simulink model "tqdtqr_rebuild_V3"  (R2021b)
settings: Solver=VariableStepAuto  StartTime=0.0  StopTime=10.0  RelTol=1e-3
undefined symbols (not defined in the file): ATQD_AfterTqMinGain_X_Deg, ATQD_APSCreepBaseTqD_X_kph, ATQD_APSCreepBaseTqD_Y_Deg, ATQD_APSCreepBaseTqR_X_kph, ATQD_APSCreepBaseTqR_Y_Deg, ATQD_APSCreepIterm_X_kph, ATQD_APSCreepIterm_Y_kph, ATQD_APSCreepPterm_X_kph, ATQD_APSCreepPterm_Y_kph, ATQD_APSDecReq_X_kph, ATQD_APSDecReq_Y_mps2, ATQD_APSDecReqCMD_X_kph, ATQD_APSDecReqTs_X_pct, ATQD_APSDecTimeGain_X_Deg, ATQD_APSDecTimeGain_Y_s, ATQD_APSReqLowSpd_X_Deg, ATQD_AutoHoldReleaseBPS_X_Deg, ATQD_AWDLoadTrqnsGain_X_kg, ATQD_AWDLoadTrqnsGain_Y_pct, ATQD_BOSEnBPSPosn_X_kph, ATQD_BOSMap_X_rpm, ATQD_BOSMap_Y_pct, ATQD_CreepBaseTqD_X_kph, ATQD_CreepBaseTqD_Y_Deg, ATQD_CreepBaseTqR_X_kph, ATQD_CreepBaseTqR_Y_Deg, ATQD_CreepBPSDisPosn_X_Deg, ATQD_CreepBPSDisPosnR_X_Deg, ATQD_CreepBPSEnPosn_X_Deg, ATQD_CreepBPSEnPosnR_X_Deg, ATQD_CreepDeltaTq_X_kph, ATQD_CreepIterm_X_kph, ATQD_CreepIterm_Y_kph, ATQD_CreepItermMaxLimit_X_pct, ATQD_CreepPreloadTime_X_kph, ATQD_CreepPreloadTq_X_kph, ATQD_CreepPreloadTq_Y_s, ATQD_CreepProtTq_X_Deg, ATQD_CreepPterm_X_kph, ATQD_CreepPterm_Y_kph, ATQD_CreepRrTqSpRat_X_rpm, ATQD_CreepRrTqSpRat_Y_Nm, ATQD_CreepTargetSpdD_X_pct, ATQD_CreepTargetSpdR_X_pct, ATQD_CreepUpLimitTq_X_rpm, ATQD_DecIneOPDHoldEnDelay_X_Deg, ATQD_DecIneOPDHoldEnDelay_Y_bar, ATQD_ECOTqMapD_X_rpm, ATQD_ECOTqMapD_Y_pct, ATQD_EMTqMapD_X_rpm, ATQD_EMTqMapD_Y_pct, ATQD_EOPDTqMapDCon_X_rpm, ATQD_EOPDTqMapDCon_Y_Deg, ATQD_EstInitVehWeight_X_c, ATQD_FAfterTqCMDGain_X_rpm, ATQD_FAfterTqCMDGain_Y_pct, ATQD_ForceLowSpd_X_Deg, ATQD_ForcePLimitSpd_X_Deg, ATQD_FrLossMAPLowV_X_rpm, ATQD_FrLossMAPLowV_Y_Nm ... (+949)
libraries: simulink x235, hcu_lib x208, tqr x63, tqd x6
(part 24 of 37)

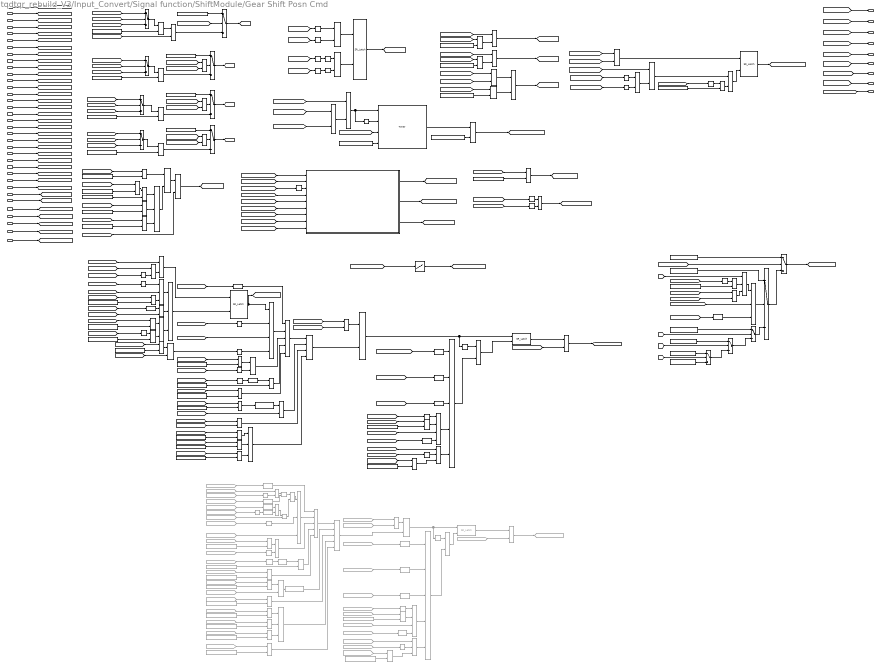
== system tqdtqr_rebuild_V3/Input_Convert/Signal function/ShiftModule/Gear Shift Posn Cmd ==
  note: Get max wheel rpm
  note: Allow D R conditions
  note: Prevent user accidental touch D to N
  note: Force P conditions
  note: Allow P N conditions
  note: Decide final gear shifter CMD
  note: Shifter value determine with DDM detection
  note: Failsafe for Shifter PButton fail
  VTQD_ShifterHandleCmd_enum : Inport
  VPMM_PowerSta_enum : Inport  Port=2
  VINP_DrDoorSW_flg : Inport  Port=3
  VVMC_APSShiftPosnReq_enum : Inport  Port=4
  VVMC_APSActive_flg : Inport  Port=5
  VINP_DriverSeatBeltCmd_flg : Inport  Port=6
  VTQD_EPBCarWashMode_flg : Inport  Port=7
  VTQD_VehActSpd_kph : Inport  Port=8
  VINP_ChrgPlugSta_enum : Inport  Port=9
  VTQD_GearActualPosn_enum : Inport  Port=10
  VTQD_AfterAvailableTqDemFr_Nm : Inport  Port=11
  VTQD_AfterAvailableTqDemRr_Nm : Inport  Port=12
  VTQR_NoABSFEDUWhlTqReq_Nm : Inport  Port=13
  VTQR_NoABSREDUWhlTqReq_Nm : Inport  Port=14
  task_time_s : Inport  Port=15
  VINP_DOASta_flg : Inport  Port=16
  VTQD_IVIPwrLock_flg : Inport  Port=17
  VTQD_BrkSwSta_flg : Inport  Port=18
  VTQD_OPDHoldAllowPark_flg : Inport  Port=19
  VINP_CAASSta_enum : Inport  Port=20
  VDDM_VCURAPSErrLv2_flg : Inport  Port=21
  VDDM_VCURAPSErrLv3_flg : Inport  Port=22
  VINP_APSStaSystem_enum : Inport  Port=23
  VDDM_Shifter1Err_flg : Inport  Port=24
  SWC_RegenUp : Inport  Port=25
  SWC_RegenDown : Inport  Port=26
  VDDM_ShifterSigErrCFS_flg : Inport  Port=27
  VTQD_ShifterFailsta_enum : Inport  Port=28
  VTQD_FrShaftSpd_rpm : Inport  Port=29
  VTQD_RrShaftSpd_rpm : Inport  Port=30
  VINP_EPBSta_enum : Inport  Port=31
  VINP_VehSpeed_kph : Inport  Port=32
  VVMC_EstSlope_Deg : Inport  Port=33
  VPMM_DrSeatSta_enum : Inport  Port=34
  VINP_ShifterHandleCmd_enum : Inport  Port=35
  AND : Logic  Commented=on  AllPortsSameDT=off  OutDataTypeStr=boolean
  AND1 : Logic  Commented=on  AllPortsSameDT=off  OutDataTypeStr=boolean
  AND{6,8..12,14..15,21..22} (10 alike) : Logic  AllPortsSameDT=off  OutDataTypeStr=boolean
  AND13 : Logic  Inputs=3  AllPortsSameDT=off  OutDataTypeStr=boolean
  AND16 : Logic  Inputs=4  AllPortsSameDT=off  OutDataTypeStr=boolean
  AND17 : Logic  Operator=OR  AllPortsSameDT=off  OutDataTypeStr=boolean
  AND18 : Logic  Inputs=4  AllPortsSameDT=off  OutDataTypeStr=boolean
  AND19 : Logic  Inputs=4  AllPortsSameDT=off  OutDataTypeStr=boolean
  AND2 : Logic  Commented=on  Inputs=4  AllPortsSameDT=off  OutDataTypeStr=boolean
  AND20 : Logic  Operator=OR  AllPortsSameDT=off  OutDataTypeStr=boolean
  AND3 : Logic  Commented=on  Operator=OR  AllPortsSameDT=off  OutDataTypeStr=boolean
  AND4 : Logic  Commented=on  Inputs=3  AllPortsSameDT=off  OutDataTypeStr=boolean
  AND5 : Logic  Commented=on  Inputs=5  AllPortsSameDT=off  OutDataTypeStr=boolean
  AND7 : Logic  Commented=on  AllPortsSameDT=off  OutDataTypeStr=boolean
  Constant : Constant  Value=ENUM_GEARSHIFTCMD_R
  Constant1 : Constant  Value=ENUM_POWERSTA_READY
  Constant10 : Constant  Value=KTQD_StandbyAllowPNSW_flg
  Constant11 : Constant  Commented=on  Value=KTQD_OPDHoldAllowGearPSW_flg
  Constant12 : Constant  Value=ENUM_SHIFTCOMMAND_D
  Constant13 : Constant  Value=ENUM_SHIFTCOMMAND_N
  Constant14 : Constant  Commented=on  Value=ENUM_CAASSTA_SHIFTGEARTOP
  Constant15 : Constant  Commented=on  Value=ENUM_PWRSTASW_READY
  Constant16 : Constant  Commented=on  Value=ENUM_SHIFTCOMMAND_P
  Constant17 : Constant  Value=ENUM_POWERSTA_STANDBY
  Constant18 : Constant  Value=ENUM_POWERSTA_ON
  Constant19 : Constant  Value=ENUM_POWERSTA_READY
  Constant2 : Constant  Value=ENUM_GEARSHIFTCMD_N
  Constant20 : Constant  Commented=on  Value=ENUM_CHRGPLUGSTA_NONE
  Constant21 : Constant  Commented=on  Value=ENUM_APSSYSTEMSTA_REMOTEACTIVE
  Constant22 : Constant  Value=ENUM_CHRGPLUGSTA_NONE
  Constant23 : Constant  Commented=on  Value=ENUM_APSSYSTEMSTA_REMOTEACTIVE
  Constant24 : Constant  Commented=on  Value=ENUM_PWRSTASW_STANDBY
  Constant25 : Constant  Commented=on  Value=ENUM_PWRSTASW_ON
  Constant26 : Constant  Commented=on  Value=ENUM_PWRSTASW_READY
  Constant27 : Constant  Value=KTQD_ShifterFail2P_s
  Constant28 : Constant  Value=KTQD_ShifterFail2P_s
  Constant29 : Constant  Value=KTQD_ForcePLimitSpd_kph
  Constant3 : Constant  Value=ENUM_GEARSHIFTCMD_P
  Constant30 : Constant  Value=ENUM_SHIFTERERRSTA_PBUTTONFAILURE
  Constant31 : Constant  Value=ENUM_SHIFTERERRSTA_HALLFAILURE
  Constant{5,32..34} (4 alike) : Constant  Value=FALSE
  Constant35 : Constant  Value=ENUM_SHIFTERERRSTA_SHIFTERFAILURE
  Constant36 : Constant  Value=ENUM_SHIFTCOMMAND_R
  Constant37 : Constant  Commented=on  Value=KTQD_ForcePLimitSpd_kph
  Constant38 : Constant  Value=KTQD_OPDHoldAllowGearPSW_flg
  Constant39 : Constant  Value=ENUM_CAASSTA_SHIFTGEARTOP
  Constant4 : Constant  Value=ENUM_GEARSHIFTCMD_D
  Constant40 : Constant  Value=ENUM_PWRSTASW_READY
  Constant41 : Constant  Value=ENUM_SHIFTCOMMAND_P
  Constant42 : Constant  Value=ENUM_CHRGPLUGSTA_NONE
  Constant43 : Constant  Value=ENUM_APSSYSTEMSTA_REMOTEACTIVE
  Constant44 : Constant  Value=ENUM_APSSYSTEMSTA_REMOTEACTIVE
  Constant45 : Constant  Value=ENUM_PWRSTASW_STANDBY
  Constant46 : Constant  Value=ENUM_PWRSTASW_ON
  Constant47 : Constant  Value=ENUM_PWRSTASW_READY
  Constant48 : Constant  Value=ENUM_EPBSTA_APPLIED
  Constant49 : Constant  Value=KTQD_DoorOpen2GearPRestSpd_kph
  Constant50 : Constant  Value=ENUM_GEARACTUALPOSN_P
  Constant6 : Constant  Value=ENUM_GEARSHIFTCMD_NONE
  Constant7 : Constant  Value=ENUM_GEARSHIFTCMD_P
  Constant8 : Constant  Value=ENUM_SHIFTCOMMAND_P
  Constant9 : Constant  Value=KTQD_DriveProtVehSpdGain_kph
  Delay : Delay  Commented=on  DelayLength=1
  Delay1 : Delay  Commented=on  DelayLength=1
  Delay{4..6,10..11} (5 alike) : Delay  DelayLength=1  InitialCondition=single(0)
      settings: AttributesFormatString=%<InitialCondition>
  Delay{2..3,7..8,12..13} (6 alike) : Delay  DelayLength=1
  Delay9 : Delay  DelayLength=1  InitialCondition=ENUM_GEARACTUALPOSN_P
      settings: AttributesFormatString=%<InitialCondition>
  Detect Change : simulink/Logic and Bit Operations/Detect Change  Commented=on  vinit=uint8(0)  OutDataTypeStr=boolean
  Detect Change1 : simulink/Logic and Bit Operations/Detect Change  Commented=on  vinit=uint8(0)  OutDataTypeStr=boolean
  Detect Change2 : simulink/Logic and Bit Operations/Detect Change  vinit=0  OutDataTypeStr=boolean
  Detect Change3 : simulink/Logic and Bit Operations/Detect Change  vinit=0  OutDataTypeStr=boolean
  Detect Change4 : simulink/Logic and Bit Operations/Detect Change  vinit=boolean(0)  OutDataTypeStr=boolean
  Detect Decrease1 : simulink/Logic and Bit Operations/Detect Decrease  Commented=on  vinit=0.0  OutDataTypeStr=boolean
  Detect Decrease2 : simulink/Logic and Bit Operations/Detect Decrease  vinit=0.0  OutDataTypeStr=boolean
  Detect Increase : simulink/Logic and Bit Operations/Detect Increase  vinit=boolean(0)  OutDataTypeStr=boolean
  Detect Increase{1..5} (5 alike) : simulink/Logic and Bit Operations/Detect Increase  Commented=on  vinit=boolean(0)  OutDataTypeStr=boolean
  Detect Increase6 : simulink/Logic and Bit Operations/Detect Increase  Commented=on  vinit=0.0  OutDataTypeStr=boolean
  Detect Increase7 : simulink/Logic and Bit Operations/Detect Increase  vinit=0.0  OutDataTypeStr=boolean
  Detect Increase8 : simulink/Logic and Bit Operations/Detect Increase  vinit=0.0  OutDataTypeStr=boolean
  Detect Increase9 : simulink/Logic and Bit Operations/Detect Increase  vinit=0.0  OutDataTypeStr=boolean
  Drive Protection : Subsystem
  Equal{,1..2,4..7,9,16..20,22..23,25..26} (17 alike) : RelationalOperator  Operator===  OutDataTypeStr=boolean  RndMeth=Simplest
  Equal{3,10,12..13,15} (5 alike) : RelationalOperator  Commented=on  Operator===  OutDataTypeStr=boolean  RndMeth=Simplest
  Equal11 : RelationalOperator  Commented=on  Operator=~=  OutDataTypeStr=boolean  RndMeth=Simplest
  Equal14 : RelationalOperator  Commented=on  Operator=~=  OutDataTypeStr=boolean  RndMeth=Simplest
  Equal21 : RelationalOperator  Operator=~=  OutDataTypeStr=boolean  RndMeth=Simplest
  Equal24 : RelationalOperator  Operator=~=  OutDataTypeStr=boolean  RndMeth=Simplest
  Equal8 : RelationalOperator  Operator=<=  OutDataTypeStr=boolean  RndMeth=Simplest
  From{27,46,53,108} (4 alike) : From  Commented=on  GotoTag=VTQD_EPBCarWashMode_flg
  From12 : From  Commented=on  GotoTag=VINP_DOASta_flg
  From13 : From  Commented=on  GotoTag=VTQD_ShifterHandleCmd_enum
  From26 : From  Commented=on  GotoTag=VTQD_IVIPwrLock_flg
  From28 : From  Commented=on  GotoTag=VVMC_APSActive_flg
  From32 : From  Commented=on  GotoTag=VTQD_OPDHoldAllowPark_flg
  From42 : From  Commented=on  GotoTag=VINP_CAASSta_enum
  From43 : From  Commented=on  GotoTag=VINP_DrDoorSW_flg
  From44 : From  Commented=on  GotoTag=VINP_SeatSW_flg
  From45 : From  Commented=on  GotoTag=VINP_DriverSeatBeltCmd_flg
  From47 : From  Commented=on  GotoTag=VTQD_VehActSpd_kph
  From48 : From  Commented=on  GotoTag=VINP_ChrgPlugSta_enum
  From{49..52} (4 alike) : From  Commented=on  GotoTag=VPMM_PowerSta_enum
  From54 : From  Commented=on  GotoTag=VINP_DrDoorSW_flg
  From55 : From  Commented=on  GotoTag=VINP_SeatSW_flg
  From56 : From  Commented=on  GotoTag=VINP_DriverSeatBeltCmd_flg
  From57 : From  Commented=on  GotoTag=VTQD_ForceP_flg
  From58 : From  Commented=on  GotoTag=VVMC_APSShiftPosnReq_enum
  From59 : From  Commented=on  GotoTag=VVMC_APSActive_flg
  From60 : From  Commented=on  GotoTag=VVMC_APSShiftPosnReq_enum
  From61 : From  Commented=on  GotoTag=VDDM_VCURAPSErrLv2_flg
  From62 : From  Commented=on  GotoTag=VDDM_VCURAPSErrLv3_flg
  From63 : From  Commented=on  GotoTag=VDDM_VCURAPSErrLv3_flg
  From64 : From  Commented=on  GotoTag=VINP_APSStaSystem_enum
  From65 : From  Commented=on  GotoTag=VINP_DOASta_flg
  From66 : From  Commented=on  GotoTag=VVMC_APSActive_flg
  From69 : From  Commented=on  GotoTag=VINP_APSStaSystem_enum
  Goto22 : Goto  Commented=on  GotoTag=VTQD_ForceP_flg
  Latch : hcu_lib/Basic_Blocks/Latch  Commented=on
  Latch1 : hcu_lib/Basic_Blocks/Latch
  Logical Operator : Logic  Commented=on  AllPortsSameDT=off  OutDataTypeStr=boolean
  Logical Operator1 : Logic  Commented=on  AllPortsSameDT=off  OutDataTypeStr=boolean
  Logical Operator{10..12,14,20,23,25,27} (8 alike) : Logic  AllPortsSameDT=off  OutDataTypeStr=boolean
      Logical Operator20 settings: AttributesFormatString=%<Operator>
  Logical Operator{8..9,13,16..19,24} (8 alike) : Logic  Operator=OR  AllPortsSameDT=off  OutDataTypeStr=boolean
      Logical Operator24 settings: AttributesFormatString=%<Operator>
  Logical Operator{5,15,21..22} (4 alike) : Logic  Operator=NOT  AllPortsSameDT=off  OutDataTypeStr=boolean
  Logical Operator2 : Logic  Inputs=3  AllPortsSameDT=off  OutDataTypeStr=boolean
  Logical Operator26 : Logic  Inputs=3  AllPortsSameDT=off  OutDataTypeStr=boolean
  Logical Operator3 : Logic  Operator=OR  Inputs=3  AllPortsSameDT=off  OutDataTypeStr=boolean
  Logical Operator4 : Logic  Commented=on  Operator=NOT  AllPortsSameDT=off  OutDataTypeStr=boolean
  Logical Operator6 : Logic  Commented=on  Inputs=3  AllPortsSameDT=off  OutDataTypeStr=boolean
  Logical Operator7 : Logic  Commented=on  AllPortsSameDT=off  OutDataTypeStr=boolean
  MTQD_ForcePLimitSpd_Y_kph : Lookup_n-D  NumberOfTableDimensions=1  BreakpointsForDimension1=ATQD_ForcePLimitSpd_X_Deg  Table=MTQD_ForcePLimitSpd_Y_kph  ExtrapMethod=Clip  InternalRulePriority=Speed  RndMeth=Simplest  InputSameDT=on
  Max : MinMax  Function=max  Inputs=2
  NOT{,2..5} (5 alike) : Logic  Commented=on  Operator=NOT  AllPortsSameDT=off  OutDataTypeStr=boolean
  NOT{1,6..12} (8 alike) : Logic  Operator=NOT  AllPortsSameDT=off  OutDataTypeStr=boolean
  OR : Logic  Operator=OR  Inputs=3  AllPortsSameDT=off  OutDataTypeStr=boolean
  OR1 : Logic  Commented=on  Operator=OR  Inputs=5  AllPortsSameDT=off  OutDataTypeStr=boolean
  OR{2,5..6,9..10} (5 alike) : Logic  Commented=on  Operator=OR  AllPortsSameDT=off  OutDataTypeStr=boolean
  OR11 : Logic  Operator=OR  Inputs=5  AllPortsSameDT=off  OutDataTypeStr=boolean
  OR{3..4,12..13} (4 alike) : Logic  Operator=OR  AllPortsSameDT=off  OutDataTypeStr=boolean
  OR14 : Logic  Operator=OR  Inputs=3  AllPortsSameDT=off  OutDataTypeStr=boolean
  OR15 : Logic  Operator=OR  Inputs=5  AllPortsSameDT=off  OutDataTypeStr=boolean
  OR16 : Logic  Operator=OR  Inputs=3  AllPortsSameDT=off  OutDataTypeStr=boolean
  OR7 : Logic  Commented=on  Operator=OR  Inputs=5  AllPortsSameDT=off  OutDataTypeStr=boolean
  OR8 : Logic  Commented=on  Operator=OR  Inputs=3  AllPortsSameDT=off  OutDataTypeStr=boolean
  Relational Operator{,6,8,10} (4 alike) : RelationalOperator  Operator===  OutDataTypeStr=boolean  RndMeth=Simplest
  Relational Operator1 : RelationalOperator  Commented=on  Operator===  OutDataTypeStr=boolean  RndMeth=Simplest
  Relational Operator2 : RelationalOperator  Commented=on  Operator=<=  OutDataTypeStr=boolean  RndMeth=Simplest
  Relational Operator3 : RelationalOperator  OutDataTypeStr=boolean  RndMeth=Simplest
  Relational Operator4 : RelationalOperator  Operator=<=  OutDataTypeStr=boolean  RndMeth=Simplest
  Relational Operator5 : RelationalOperator  Commented=on  Operator=~=  OutDataTypeStr=boolean  RndMeth=Simplest
  Relational Operator7 : RelationalOperator  Operator=<=  OutDataTypeStr=boolean  RndMeth=Simplest
  Relational Operator9 : RelationalOperator  Operator=>  OutDataTypeStr=boolean  RndMeth=Simplest
  SR_Latch{,2..4} (4 alike) : hcu_lib/Basic_Blocks/SR_Latch
  SR_Latch1 : hcu_lib/Basic_Blocks/SR_Latch  Commented=on
  Switch{,1..12} (13 alike) : Switch  Criteria=u2 ~= 0
      settings: AttributesFormatString=%<Criteria>
  Timer : hcu_lib/Basic_Blocks/Timer
  VTQD_GearShiftCMD_enum : Outport
  VTQD_PwrStaAllowPN_flg : Outport  Port=2
  VTQD_PwrStaAllowDR_flg : Outport  Port=3
  VTQD_DriveProtRemove_flg : Outport  Port=4
  VTQD_DriveProtEn_flg : Outport  Port=5
  VTQD_ForceP_flg : Outport  Port=6
  VTQD_MaxShaftSpd_rpm : Outport  Port=7
  VTQD_DOALatchReq_flg : Outport  Port=8
  VTQD_ForcePLimitSpd_kph : Outport  Port=9
  wires:
  Switch2/1 -> Switch4/3
  Constant2/1 -> Switch4/1
  Switch1/1 -> Switch2/3
  [P] -> Switch2/2
  Constant3/1 -> Switch2/1
  Switch3/1 -> Switch1/3
  Constant/1 -> Switch3/1
  Constant4/1 -> Switch1/1
  [R] -> Switch3/2
  [D] -> Switch1/2
  VTQD_ShifterHandleCmd_enum/1 -> [VTQD_ShifterHandleCmd_enum]
  VPMM_PowerSta_enum/1 -> [VPMM_PowerSta_enum]
  [VPMM_PowerSta_enum] -> Equal7/1
  Constant1/1 -> Equal7/2
  Constant6/1 -> Switch3/3
  Switch4/1 -> Switch/3
  VINP_DrDoorSW_flg/1 -> [VINP_DrDoorSW_flg]
  [VTQD_ForceP_flg] -> Switch/2
  Constant7/1 -> Switch/1
  VVMC_APSShiftPosnReq_enum/1 -> [VVMC_APSShiftPosnReq_enum]
  VVMC_APSActive_flg/1 -> [VVMC_APSActive_flg]
  VINP_DriverSeatBeltCmd_flg/1 -> [VINP_DriverSeatBeltCmd_flg]
  VTQD_EPBCarWashMode_flg/1 -> [VTQD_EPBCarWashMode_flg]
  VINP_ChrgPlugSta_enum/1 -> [VINP_ChrgPlugSta_enum]
  VTQR_NoABSREDUWhlTqReq_Nm/1 -> [VTQR_NoABSREDUWhlTqReq_Nm]
  VTQD_AfterAvailableTqDemFr_Nm/1 -> [VTQD_AfterAvailableTqDemFr_Nm]
  VTQD_GearActualPosn_enum/1 -> [VTQD_GearActualPosn_enum]
  VTQR_NoABSFEDUWhlTqReq_Nm/1 -> [VTQR_NoABSFEDUWhlTqReq_Nm]
  VTQD_AfterAvailableTqDemRr_Nm/1 -> [VTQD_AfterAvailableTqDemRr_Nm]
  task_time_s/1 -> [task_time_s]
  VINP_DOASta_flg/1 -> [VINP_DOASta_flg]
  Constant9/1 -> Equal8/2
  [VTQD_VehActSpd_kph] -> Delay11/1
  [VTQD_EPBCarWashMode_flg] -> Detect Increase/1
  Detect Increase/1 -> Logical Operator3/3
  [N] -> Logical Operator2/1
  Logical Operator2/1 -> Logical Operator3/1
  Logical Operator3/1 -> Switch4/2
  [task_time_s] -> Drive Protection/8(task_time_s)  "task_time_s"
  [VTQD_VehActSpd_kph] -> Delay6/1
  [VTQD_AfterAvailableTqDemRr_Nm] -> Drive Protection/7(VTQD_AfterAvailableTqDemRr_Nm)
  [VTQD_AfterAvailableTqDemFr_Nm] -> Drive Protection/4(VTQD_AfterAvailableTqDemFr_Nm)
  [VTQR_NoABSREDUWhlTqReq_Nm] -> Drive Protection/5(VTQR_NoABSREDUWhlTqReq_Nm)
  [VTQR_NoABSFEDUWhlTqReq_Nm] -> Drive Protection/6(VTQR_NoABSFEDUWhlTqReq_Nm)
  [VTQD_ShifterHandleCmd_enum] -> Drive Protection/1(VTQD_ShifterHandleCmd_enum)
  Drive Protection/2(VTQD_DriveProtToPsnN_flg) -> [VTQD_DriveProtToPsnN_flg]
  [VTQD_GearActualPosn_enum] -> Drive Protection/2(VTQD_GearActualPosn_enum)
  VTQD_IVIPwrLock_flg/1 -> [VTQD_IVIPwrLock_flg]
  [VTQD_DriveProtToPsnN_flg] -> Logical Operator3/2
  Equal8/1 -> Logical Operator2/2
  VTQD_BrkSwSta_flg/1 -> [VTQD_BrkSwSta_flg]
  [VTQD_BrkSwSta_flg] -> Drive Protection/9(VTQD_BrkSwSta_flg)
  OR3/1 -> Logical Operator2/3
  [VTQD_BrkSwSta_flg] -> OR3/1
  [VVMC_APSActive_flg] -> OR3/2
  VTQD_OPDHoldAllowPark_flg/1 -> [VTQD_OPDHoldAllowPark_flg]
  VINP_CAASSta_enum/1 -> [VINP_CAASSta_enum]
  VDDM_VCURAPSErrLv3_flg/1 -> [VDDM_VCURAPSErrLv3_flg]
  VINP_APSStaSystem_enum/1 -> [VINP_APSStaSystem_enum]
  VDDM_VCURAPSErrLv2_flg/1 -> [VDDM_VCURAPSErrLv2_flg]
  Constant8/1 -> Equal/2
  Equal1/1 -> Switch9/3
  Switch8/1 -> Equal2/1
  Switch10/1 -> [P]
  [ShifterHall_Fail] -> Logical Operator17/1
  Constant33/1 -> Switch11/1
  [VVMC_APSShiftPosnReq_enum] -> Switch6/1
  [VVMC_APSActive_flg] -> Switch7/2
  [Shifter_Fail] -> Logical Operator18/2
  Switch12/1 -> [N]
  Constant13/1 -> Equal9/2
  [VVMC_APSActive_flg] -> Switch8/2
  [VVMC_APSShiftPosnReq_enum] -> Switch8/1
  [VVMC_APSActive_flg] -> Switch6/2
  Equal9/1 -> Switch12/3
  Logical Operator8/1 -> Switch9/2
  [Shifter_Fail] -> Logical Operator17/2
  Switch7/1 -> Equal9/1
  [VTQD_ShifterHandleCmd_enum] -> Switch5/3
  Constant5/1 -> Switch10/1
  Switch11/1 -> [D]
  [VVMC_APSShiftPosnReq_enum] -> Switch5/1
  Equal2/1 -> Switch11/3
  [VTQD_ShifterHandleCmd_enum] -> Switch6/3
  [VVMC_APSShiftPosnReq_enum] -> Switch7/1
  Constant12/1 -> Equal2/2
  Switch5/1 -> Equal/1
  Constant32/1 -> Switch9/1
  [ShifterHall_Fail] -> Logical Operator8/1
  Switch9/1 -> [R]
  Constant36/1 -> Equal1/2
  [VTQD_ShifterFail2P_flg] -> Logical Operator19/2
  [VTQD_ShifterHandleCmd_enum] -> Switch8/3
  [ShifterHall_Fail] -> Logical Operator18/1
  [VTQD_ShifterHandleCmd_enum] -> Switch7/3
  Equal/1 -> Logical Operator19/1
  Logical Operator19/1 -> Switch10/3
  Constant34/1 -> Switch12/1
  Logical Operator18/1 -> Switch12/2
  [VTQD_ShifterPBackUpCmd_flg] -> Switch10/2
  Switch6/1 -> Equal1/1
  [Shifter_Fail] -> Logical Operator8/2
  Logical Operator17/1 -> Switch11/2
  [VVMC_APSActive_flg] -> Switch5/2
  Logical Operator15/1 -> Timer/2
  [Shifter_Fail] -> Logical Operator16/2
  SR_Latch/1 -> [PRESS_BOTH]
  Constant29/1 -> Relational Operator4/2
  Logical Operator22/1 -> Logical Operator20/2
  AND9/1 -> SR_Latch/2
  Logical Operator13/1 -> Logical Operator14/1
  [VDDM_ShifterSigErrCFS_flg] -> Logical Operator12/1
  [VDDM_Shifter1Err_flg] -> Logical Operator13/2
  Logical Operator21/1 -> Logical Operator20/1
  Logical Operator14/1 -> [Shifter_Fail]
  NOT7/1 -> AND9/2
  [task_time_s] -> Timer/3
  Relational Operator3/1 -> [VTQD_ShifterFail2P_flg]  "VTQD_ShifterFail2P_flg"
  [PRESS_BOTH] -> Logical Operator10/1
  Constant31/1 -> Equal19/2
  Logical Operator20/1 -> Logical Operator24/2
  [PRESS_BOTH] -> Logical Operator24/1
  Logical Operator12/1 -> [ShifterHall_Fail]
  [Shifter_Fail] -> Logical Operator9/1
  [VTQD_ShifterFailsta_enum] -> Equal18/1
  Logical Operator16/1 -> SR_Latch3/1
  Logical Operator23/1 -> SR_Latch3/2
  Logical Operator24/1 -> Logical Operator23/1
  Relational Operator4/1 -> Logical Operator23/2
  [SWC_RegenDown] -> Delay3/1
  [ShifterPButton_Fail] -> Logical Operator9/2
  Constant27/1 -> Timer/4
  Equal18/1 -> Logical Operator11/2
  Equal19/1 -> Logical Operator12/2
  [VDDM_ShifterSigErrCFS_flg] -> Logical Operator13/1
  [VDDM_ShifterSigErrCFS_flg] -> Logical Operator11/1
  AND8/1 -> SR_Latch/1
  Constant28/1 -> Relational Operator3/2
  Constant30/1 -> Equal18/2
  Timer/1 -> Relational Operator3/1
  Equal20/1 -> Logical Operator14/2
  Logical Operator9/1 -> Logical Operator10/2
  SR_Latch3/1 -> [VTQD_ShifterPBackUpCmd_flg]
  [ShifterPButton_Fail] -> Logical Operator16/1
  Logical Operator11/1 -> [ShifterPButton_Fail]
  [SWC_RegenUp] -> Delay2/1
  [VTQD_ShifterFailsta_enum] -> Equal19/1
  Constant35/1 -> Equal20/2
  [VTQD_VehActSpd_kph] -> Delay10/1
  NOT6/1 -> AND9/1
  [VTQD_ShifterFailsta_enum] -> Equal20/1
  Logical Operator10/1 -> Logical Operator15/1, Timer/1
  [VDDM_Shifter1Err_flg] -> Logical Operator22/1
  [VDDM_ShifterSigErrCFS_flg] -> Logical Operator21/1
  VDDM_ShifterSigErrCFS_flg/1 -> [VDDM_ShifterSigErrCFS_flg]
  SWC_RegenUp/1 -> [SWC_RegenUp]
  SWC_RegenDown/1 -> [SWC_RegenDown]
  VDDM_Shifter1Err_flg/1 -> [VDDM_Shifter1Err_flg]
  VTQD_ShifterFailsta_enum/1 -> [VTQD_ShifterFailsta_enum]
  Switch/1 -> [VTQD_GearShiftCMD_enum]  "VTQD_GearShiftCMD_enum"
  [VTQD_GearShiftCMD_enum] -> VTQD_GearShiftCMD_enum/1
  Equal7/1 -> [VTQD_PwrStaAllowDR_flg]  "VTQD_PwrStaAllowDR_flg"
  [VTQD_PwrStaAllowDR_flg] -> VTQD_PwrStaAllowDR_flg/1
  [VTQD_PwrStaAllowPN_flg] -> VTQD_PwrStaAllowPN_flg/1
  Drive Protection/1(VTQD_DriveProtRemove_flg) -> [VTQD_DriveProtRemove_flg]
  [VTQD_DriveProtRemove_flg] -> VTQD_DriveProtRemove_flg/1
  Drive Protection/3(VTQD_DriveProtEn_flg) -> [VTQD_DriveProtEn_flg]
  [VTQD_DriveProtEn_flg] -> VTQD_DriveProtEn_flg/1
  [VTQD_ForceP_flg] -> VTQD_ForceP_flg/1
  Max/1 -> [VTQD_MaxShaftSpd_rpm]  "VTQD_MaxShaftSpd_rpm"
  [VTQD_FrShaftSpd_rpm] -> Delay4/1
  Delay4/1 -> Max/1
  [VTQD_RrShaftSpd_rpm] -> Delay5/1
  Delay5/1 -> Max/2
  VTQD_FrShaftSpd_rpm/1 -> [VTQD_FrShaftSpd_rpm]
  VTQD_RrShaftSpd_rpm/1 -> [VTQD_RrShaftSpd_rpm]
  [VTQD_MaxShaftSpd_rpm] -> VTQD_MaxShaftSpd_rpm/1
  From62/1 -> Logical Operator7/2
  Delay1/1 -> AND2/1
  Logical Operator6/1 -> OR1/5
  AND5/1 -> AND3/2
  Logical Operator7/1 -> AND3/1
  Constant20/1 -> Equal14/2
  Delay/1 -> Detect Increase6/1
  Relational Operator2/1 -> AND5/3
  From47/1 -> Relational Operator2/1
  From32/1 -> Delay/1
  Equal10/1 -> OR7/5
  NOT4/1 -> AND4/2
  Constant15/1 -> Equal3/2
  From55/1 -> NOT5/1
  OR8/1 -> AND5/4
  From50/1 -> Equal3/1
  Constant24/1 -> Equal15/2
  OR2/1 -> Goto22/1  "VTQD_ForceP_flg"
  SR_Latch1/1 -> OR2/1
  OR10/1 -> AND4/1
  From12/1 -> AND4/3
  Logical Operator/1 -> OR10/1
  OR7/1 -> AND5/1
  Detect Increase6/1 -> AND/1
  From48/1 -> Equal14/1
  Detect Decrease1/1 -> OR7/1
  NOT3/1 -> OR6/2
  From51/1 -> Equal12/1
  From52/1 -> Equal13/1
  Equal12/1 -> OR8/2
  From43/1 -> Detect Increase1/1
  Constant25/1 -> Equal12/2
  Equal15/1 -> OR8/1
  AND4/1 -> OR7/2
  AND3/1 -> SR_Latch1/1, NOT/1
  Detect Change/1 -> OR1/1
  NOT/1 -> AND1/1
  From63/1 -> Logical Operator4/1
  Detect Increase1/1 -> Logical Operator/2
  NOT2/1 -> AND7/2
  Equal14/1 -> AND7/1
  AND7/1 -> OR7/3
  Constant26/1 -> Equal13/2
  Logical Operator4/1 -> Logical Operator6/2
  Logical Operator1/1 -> OR10/2
  OR1/1 -> AND1/2
  Relational Operator1/1 -> Logical Operator6/3
  Detect Change1/1 -> AND2/4
  Constant16/1 -> Equal11/2
  Detect Increase5/1 -> OR1/3
  Equal11/1 -> AND2/2
  Equal13/1 -> OR8/3
  Constant37/1 -> Relational Operator2/2
  From13/1 -> Detect Change/1
  AND2/1 -> OR1/4
  From61/1 -> Logical Operator6/1
  From108/1 -> NOT2/1
  From49/1 -> Equal15/1
  From28/1 -> Detect Increase5/1
  From53/1 -> Detect Decrease1/1
  Constant11/1 -> AND/2
  AND1/1 -> SR_Latch1/2
  NOT5/1 -> Detect Increase3/1
  OR9/1 -> Logical Operator1/1
  From59/1 -> AND2/3
  From66/1 -> Logical Operator7/1
  From42/1 -> Equal10/1
  From58/1 -> Equal11/1
  Detect Increase2/1 -> OR9/1
  From56/1 -> Detect Increase2/1
  From57/1 -> Delay1/1
  From44/1 -> NOT3/1
  From27/1 -> Detect Increase4/1
  From46/1 -> NOT4/1
  Latch/1 -> AND5/2
  Constant21/1 -> Relational Operator5/2
  From54/1 -> Logical Operator1/2
  OR6/1 -> Logical Operator/1
  Constant23/1 -> Relational Operator1/2
  Detect Increase3/1 -> OR9/2
  From69/1 -> Relational Operator1/1
  From64/1 -> Relational Operator5/1
  OR5/1 -> Latch/1
  Equal3/1 -> OR5/1
  Relational Operator5/1 -> AND5/5
  From26/1 -> OR2/2
  Detect Increase4/1 -> OR1/2
  Constant14/1 -> Equal10/2
  From45/1 -> OR6/1
  From65/1 -> OR5/2
  From60/1 -> Detect Change1/1
  AND/1 -> OR7/4
  VTQD_VehActSpd_kph/1 -> [VTQD_VehActSpd_kph]
  OR4/1 -> [VTQD_PwrStaAllowPN_flg]  "VTQD_PwrStaAllowPN_flg"
  [VPMM_PowerSta_enum] -> Equal5/1
  Constant19/1 -> Equal6/2
  Equal6/1 -> OR/3
  Equal16/1 -> AND6/1
  Constant22/1 -> Equal16/2
  AND12/1 -> OR/1
  Equal4/1 -> AND12/1
  AND6/1 -> OR4/1
  [VINP_ChrgPlugSta_enum] -> Equal16/1
  Constant17/1 -> Equal4/2
  [VPMM_PowerSta_enum] -> Equal6/1
  Constant10/1 -> AND12/2
  [VTQD_EPBCarWashMode_flg] -> OR4/2
  [VPMM_PowerSta_enum] -> Equal4/1
  Constant18/1 -> Equal5/2
  Equal5/1 -> OR/2
  OR/1 -> AND6/2
  AND13/1 -> OR14/1
  Constant49/1 -> Relational Operator9/2
  AND14/1 -> OR14/2
  [VPMM_DrSeatSta_enum] -> NOT12/1
  AND20/1 -> AND19/2
  [VTQD_EPBCarWashMode_flg] -> Detect Increase7/1
  Constant48/1 -> Relational Operator8/2
  SR_Latch4/1 -> OR12/1
  Detect Change4/1 -> AND14/1
  [VINP_APSStaSystem_enum] -> Relational Operator6/1
  [VINP_ShifterHandleCmd_enum] -> Detect Change4/1
  AND11/1 -> SR_Latch4/2
  OR13/1 -> AND22/2
  AND16/1 -> OR11/4
  Delay8/1 -> AND16/1
  AND22/1 -> SR_Latch2/1
  [VINP_DrDoorSW_flg] -> AND22/1
  OR14/1 -> SR_Latch2/2
  [VTQD_EPBCarWashMode_flg] -> NOT9/1
  Equal24/1 -> AND21/1
  Detect Increase8/1 -> OR11/3
  AND21/1 -> OR15/3
  Relational Operator/1 -> Logical Operator25/1
  Detect Increase9/1 -> AND10/1
  [VINP_ChrgPlugSta_enum] -> Equal24/1
  Relational Operator10/1 -> AND15/2
  [VVMC_APSShiftPosnReq_enum] -> Equal21/1
  Relational Operator8/1 -> AND15/1
  NOT11/1 -> AND18/2
  [VVMC_APSActive_flg] -> Detect Increase8/1
  Latch1/1 -> AND20/1
  [VTQD_EPBCarWashMode_flg] -> NOT11/1
  Constant50/1 -> Relational Operator10/2
  NOT9/1 -> AND21/2
  [VINP_DriverSeatBeltCmd_flg] -> OR13/1
  Delay9/1 -> Relational Operator10/1
  NOT12/1 -> OR13/2
  [VTQD_ForcePLimitSpd_kph] -> Relational Operator7/2
  Relational Operator7/1 -> AND19/3
  Relational Operator9/1 -> AND13/3
  [VINP_EPBSta_enum] -> Relational Operator8/1
  [VTQD_ShifterHandleCmd_enum] -> Detect Change2/1
  OR11/1 -> AND11/2
  Equal25/1 -> OR16/1
  OR16/1 -> AND19/4
  Constant42/1 -> Equal24/2
  Equal22/1 -> OR16/2
  Logical Operator26/1 -> OR11/5
  AND15/1 -> OR14/3
  OR15/1 -> AND19/1
  Detect Increase7/1 -> OR11/2
  [VINP_VehSpeed_kph] -> Relational Operator7/1
  [VINP_DrDoorSW_flg] -> NOT10/1
  Constant40/1 -> Equal26/2
  Equal26/1 -> Latch1/1
  Detect Change2/1 -> OR11/1
  [VTQD_ForceP_flg] -> Delay8/1
  [VDDM_VCURAPSErrLv3_flg] -> Logical Operator27/2
  [VPMM_PowerSta_enum] -> Equal23/1
  [VTQD_OPDHoldAllowPark_flg] -> Delay7/1
  [VINP_VehSpeed_kph] -> Relational Operator9/1
  [VDDM_VCURAPSErrLv2_flg] -> Logical Operator25/2
  SR_Latch2/1 -> AND18/1, [VTQD_DOALatchReq_flg]  "VTQD_DOALatchReq_flg"
  Constant44/1 -> Relational Operator6/2
  [VPMM_PowerSta_enum] -> Equal25/1
  [VINP_DOASta_flg] -> AND20/2
  Constant43/1 -> Relational Operator/2
  Constant39/1 -> Equal17/2
  AND18/1 -> OR15/2
  Equal17/1 -> OR15/5
  [VINP_DOASta_flg] -> AND18/3
  [VINP_CAASSta_enum] -> Equal17/1
  Constant38/1 -> AND10/2
  Logical Operator25/1 -> NOT8/1
  NOT8/1 -> AND18/4
  [VDDM_VCURAPSErrLv2_flg] -> Logical Operator26/1
  Detect Change3/1 -> AND16/4
  Delay7/1 -> Detect Increase9/1
  Equal21/1 -> AND16/2
  [VDDM_VCURAPSErrLv3_flg] -> Logical Operator5/1
  Equal23/1 -> OR16/3
  NOT1/1 -> AND11/1
  Relational Operator6/1 -> Logical Operator26/3
  NOT10/1 -> AND13/1
  Constant45/1 -> Equal25/2
  [VVMC_APSActive_flg] -> AND16/3
  Constant41/1 -> Equal21/2
  Logical Operator5/1 -> Logical Operator26/2
  [VTQD_GearActualPosn_enum] -> Delay9/1
  [VVMC_APSActive_flg] -> Logical Operator27/1
  [VTQD_BrkSwSta_flg] -> AND14/2
  OR12/1 -> [VTQD_ForceP_flg]  "VTQD_ForceP_flg"
  Detect Decrease2/1 -> OR15/1
  AND10/1 -> OR15/4
  AND19/1 -> AND17/2
  [VPMM_DrSeatSta_enum] -> AND13/2
  Logical Operator27/1 -> AND17/1
  [VTQD_IVIPwrLock_flg] -> OR12/2
  Constant47/1 -> Equal23/2
  [VPMM_PowerSta_enum] -> Equal26/1
  [VTQD_EPBCarWashMode_flg] -> Detect Decrease2/1
  [VVMC_APSShiftPosnReq_enum] -> Detect Change3/1
  [VPMM_PowerSta_enum] -> Equal22/1
  [VINP_APSStaSystem_enum] -> Relational Operator/1
  Constant46/1 -> Equal22/2
  AND17/1 -> SR_Latch4/1, NOT1/1
  VINP_EPBSta_enum/1 -> [VINP_EPBSta_enum]
  VINP_VehSpeed_kph/1 -> [VINP_VehSpeed_kph]
  MTQD_ForcePLimitSpd_Y_kph/1 -> [VTQD_ForcePLimitSpd_kph]  "VTQD_ForcePLimitSpd_kph"
  [VVMC_EstSlope_Deg] -> MTQD_ForcePLimitSpd_Y_kph/1
  VVMC_EstSlope_Deg/1 -> [VVMC_EstSlope_Deg]
  VPMM_DrSeatSta_enum/1 -> [VPMM_DrSeatSta_enum]
  [VTQD_DOALatchReq_flg] -> VTQD_DOALatchReq_flg/1
  [VTQD_ForcePLimitSpd_kph] -> VTQD_ForcePLimitSpd_kph/1
  VINP_ShifterHandleCmd_enum/1 -> [VINP_ShifterHandleCmd_enum]
  Delay6/1 -> Drive Protection/3(VTQD_VehActSpd_kph)
  Delay10/1 -> Relational Operator4/1
  Delay11/1 -> Equal8/1
  Delay2/1 -> AND8/1
  Delay12/1 -> NOT6/1
  [SWC_RegenUp] -> Delay12/1
  Delay3/1 -> AND8/2
  Delay13/1 -> NOT7/1
  [SWC_RegenDown] -> Delay13/1

== system tqdtqr_rebuild_V3/Input_Convert/Signal function/ShiftModule/SR_Latch1 ==
  set : Inport
  reset : Inport  Port=2
  Logical Operator : Logic  AllPortsSameDT=off  OutDataTypeStr=boolean
  Logical Operator1 : Logic  Operator=NOT  AllPortsSameDT=off  OutDataTypeStr=boolean
  Switch1 : Switch  Criteria=u2 ~= 0  Threshold=0.5
      settings: AttributesFormatString=<Criteria=%<Criteria>>
  Switch2 : Switch  Criteria=u2 ~= 0  Threshold=0.5
      settings: AttributesFormatString=<Criteria=%<Criteria>>
  Unit Delay : UnitDelay  SampleTime=-1  HasFrameUpgradeWarning=on
  latched : Outport
  wires:
  Switch1/1 -> Unit Delay/1, latched/1
  set/1 -> Switch1/1, Logical Operator/1
  reset/1 -> Switch2/2, Logical Operator1/1
  Unit Delay/1 -> Switch2/3
  Switch2/1 -> Switch1/3
  Logical Operator/1 -> Switch1/2
  Logical Operator1/1 -> Logical Operator/2, Switch2/1

== system tqdtqr_rebuild_V3/Input_Convert/Signal function/VehWeightEst/Calaulation ==
  task_time_s : Inport
  VTQD_VehWeightEstEn_flg : Inport  Port=2
  VTQD_VehWeightEstDis_flg : Inport  Port=3
  VTQD_VehWeightEstEnd_flg : Inport  Port=4
  VVMC_LongAcc_Gps : Inport  Port=5
  VINP_FrEDURealTMTq_Nm : Inport  Port=6
  VINP_RrEDURealTMTq_Nm : Inport  Port=7
  VINP_VehSpeed_kph : Inport  Port=8
  Front Wheel Torque : Subsystem
  Long Acc : Subsystem
  Rear Wheel Torque : Subsystem
  Vehicle Weight : Subsystem
  VTQD_EstLongAccCheckPass_flg : Outport
  VTQD_EstFrRealTqCheckPass_flg : Outport  Port=2
  VTQD_EstRrRealTqCheckPass_flg : Outport  Port=3
  VTQD_EstVehWeight_kg : Outport  Port=4
  wires:
  task_time_s/1 -> [task_time_s]
  VTQD_VehWeightEstEn_flg/1 -> [VTQD_VehWeightEstEn_flg]
  [VVMC_LongAcc_Gps] -> Long Acc/1(VVMC_LongAcc_Gps)
  [VTQD_VehWeightEstEn_flg] -> Long Acc/2(VTQD_VehWeightEstEn_flg)
  [VTQD_VehWeightEstDis_flg] -> Long Acc/3(VTQD_VehWeightEstDis_flg)
  [VTQD_VehWeightEstEnd_flg] -> Long Acc/4(VTQD_VehWeightEstEnd_flg)
  [task_time_s] -> Long Acc/5(task_time_s)
  [VINP_FrEDURealTMTq_Nm] -> Front Wheel Torque/1(VINP_FrEDURealTMTq_Nm)
  [VTQD_VehWeightEstEn_flg] -> Front Wheel Torque/2(VTQD_VehWeightEstEn_flg)
  [VTQD_VehWeightEstDis_flg] -> Front Wheel Torque/3(VTQD_VehWeightEstDis_flg)
  [VTQD_VehWeightEstEnd_flg] -> Front Wheel Torque/4(VTQD_VehWeightEstEnd_flg)
  [task_time_s] -> Front Wheel Torque/5(task_time_s)
  [VINP_RrEDURealTMTq_Nm] -> Rear Wheel Torque/1(VINP_RrEDURealTMTq_Nm)
  [VTQD_VehWeightEstEn_flg] -> Rear Wheel Torque/2(VTQD_VehWeightEstEn_flg)
  [VTQD_VehWeightEstDis_flg] -> Rear Wheel Torque/3(VTQD_VehWeightEstDis_flg)
  [VTQD_VehWeightEstEnd_flg] -> Rear Wheel Torque/4(VTQD_VehWeightEstEnd_flg)
  [task_time_s] -> Rear Wheel Torque/5(task_time_s)
  VTQD_VehWeightEstDis_flg/1 -> [VTQD_VehWeightEstDis_flg]
  VTQD_VehWeightEstEnd_flg/1 -> [VTQD_VehWeightEstEnd_flg]
  VVMC_LongAcc_Gps/1 -> [VVMC_LongAcc_Gps]
  VINP_FrEDURealTMTq_Nm/1 -> [VINP_FrEDURealTMTq_Nm]
  VINP_RrEDURealTMTq_Nm/1 -> [VINP_RrEDURealTMTq_Nm]
  Long Acc/1(VTQD_EstLongAccAvg_Gps) -> [VTQD_EstLongAccAvg_Gps]
  Long Acc/2(VTQD_EstLongAccCheckPass_flg) -> [VTQD_EstLongAccCheckPass_flg]
  Front Wheel Torque/1(VTQD_EstFrRealTqAvg_Nm) -> [VTQD_EstFrRealTqAvg_Nm]
  Front Wheel Torque/2(VTQD_EstFrRealTqCheckPass_flg) -> [VTQD_EstFrRealTqCheckPass_flg]
  Rear Wheel Torque/1(VTQD_EstRrRealTqAvg_Nm) -> [VTQD_EstRrRealTqAvg_Nm]
  Rear Wheel Torque/2(VTQD_EstRrRealTqCheckPass_flg) -> [VTQD_EstRrRealTqCheckPass_flg]
  [VTQD_EstLongAccCheckPass_flg] -> VTQD_EstLongAccCheckPass_flg/1
  [VTQD_EstRrRealTqCheckPass_flg] -> VTQD_EstRrRealTqCheckPass_flg/1
  [VTQD_EstFrRealTqCheckPass_flg] -> VTQD_EstFrRealTqCheckPass_flg/1
  [VTQD_EstFrRealTqAvg_Nm] -> Vehicle Weight/1(VTQD_EstFrRealTqAvg_Nm)
  [VTQD_EstRrRealTqAvg_Nm] -> Vehicle Weight/2(VTQD_EstRrRealTqAvg_Nm)
  [VTQD_EstLongAccAvg_Gps] -> Vehicle Weight/3(VTQD_EstLongAccAvg_Gps)
  [VINP_VehSpeed_kph] -> Vehicle Weight/4(VINP_VehSpeed_kph)
  VINP_VehSpeed_kph/1 -> [VINP_VehSpeed_kph]
  Vehicle Weight/1(VTQD_EstVehWeight_kg) -> [VTQD_EstVehWeight_kg]
  [VTQD_EstVehWeight_kg] -> VTQD_EstVehWeight_kg/1

== system tqdtqr_rebuild_V3/Input_Convert/Signal function/VehWeightEst/Condition ==
  VTQD_AfterAvailableTqDemRr_Nm : Inport
  VTQR_NoABSREDUWhlTqReq_Nm : Inport  Port=2
  VTQR_NoABSFEDUWhlTqReq_Nm : Inport  Port=3
  VTQD_AfterAvailableTqDemFr_Nm : Inport  Port=4
  VTQD_GearActualPosn_enum : Inport  Port=5
  VINP_VehSpeed_kph : Inport  Port=6
  VTQD_RollRegenDisableReq_flg : Inport  Port=7
  VINP_RegenMode_enum : Inport  Port=8
  VTQD_LowIdleAccPedal_flg : Inport  Port=9
  VTQD_BrkSwSta_flg : Inport  Port=10
  VINP_RrRBCActive_flg : Inport  Port=11
  VINP_FrRBCActive_flg : Inport  Port=12
  VINP_GRADE_Deg : Inport  Port=13
  task_time_s : Inport  Port=14
  VTQD_VehWeightEstEnd_flg : Inport  Port=15
  AND1 : Logic  Inputs=13  AllPortsSameDT=off  OutDataTypeStr=boolean
  Abs : Abs
  Abs1 : Abs
  Abs2 : Abs
  Add : Sum  Inputs=+-
  Add1 : Sum  Inputs=+-
  Constant1 : Constant  Value=KTQD_VehWeightEstSpdEnLow_kph
  Constant10 : Constant  Value=eps
  Constant11 : Constant  Value=KTQD_VehWeightEstSpdEnUp_kph
  Constant2 : Constant  Value=ENUM_REGENLEVEL_LV1
  Constant3 : Constant  Value=KTQD_RrTqDeviation_Nm
  Constant4 : Constant  Value=KTQD_FrTqDeviation_Nm
  Constant5 : Constant  Value=KTQD_VehWeightEstGradeEn_Deg
  Constant6 : Constant  Value=KTQD_VehWeighEstTime_s
  Constant7 : Constant  Value=KTQD_EstDelayEnTime_s
  Constant8 : Constant  Value=KTQD_EstWeighResetTime_s
  Constant9 : Constant  Value=ENUM_GEARACTUALPOSN_D
  Delay : Delay  DelayLength=1  InitialCondition=boolean(0)
      settings: AttributesFormatString=%<InitialCondition>
  Delay{1..4} (4 alike) : Delay  DelayLength=1  InitialCondition=single(0.0)
      settings: AttributesFormatString=%<InitialCondition>
  Delay5 : Delay  DelayLength=1
  DelayEnable : hcu_lib/Basic_Blocks/DelayEnable
  Detect Increase : simulink/Logic and Bit Operations/Detect Increase  vinit=boolean(0)  OutDataTypeStr=boolean
  Equal : RelationalOperator  Operator=<  OutDataTypeStr=boolean  RndMeth=Simplest
  Equal1 : RelationalOperator  Operator===  OutDataTypeStr=boolean  RndMeth=Simplest
  Equal2 : RelationalOperator  Operator=~=  OutDataTypeStr=boolean  RndMeth=Simplest
  Less Than1 : RelationalOperator  Operator=<  OutDataTypeStr=boolean  RndMeth=Simplest
  Less Than2 : RelationalOperator  Operator=>  OutDataTypeStr=boolean  RndMeth=Simplest
  Less Than3 : RelationalOperator  Operator=<=  OutDataTypeStr=boolean  RndMeth=Simplest
  Less Than4 : RelationalOperator  Operator=<=  OutDataTypeStr=boolean  RndMeth=Simplest
  Less Than5 : RelationalOperator  Operator=<=  OutDataTypeStr=boolean  RndMeth=Simplest
  NOT{,1..5} (6 alike) : Logic  Operator=NOT  AllPortsSameDT=off  OutDataTypeStr=boolean
  Relational Operator : RelationalOperator  OutDataTypeStr=boolean  RndMeth=Simplest
  Relational Operator1 : RelationalOperator  OutDataTypeStr=boolean  RndMeth=Simplest
  SR_Latch : hcu_lib/Basic_Blocks/SR_Latch
  Timer : hcu_lib/Basic_Blocks/Timer
  Timer1 : hcu_lib/Basic_Blocks/Timer
  VTQD_VehWeightEstEn_flg : Outport
  VTQD_VehWeightEstDis_flg : Outport  Port=2
  wires:
  Constant9/1 -> Equal1/2
  Less Than1/1 -> AND1/2  "VTQD_VehWeightEstEnCon2_flg"
  Abs/1 -> [VTQD_RrTqErr_Nm]  "VTQD_RrTqErr_Nm"
  Equal1/1 -> AND1/1  "VTQD_VehWeightEstEnCon1_flg"
  Constant11/1 -> Less Than1/2
  [VTQR_NoABSFEDUWhlTqReq_Nm] -> Delay1/1
  Constant4/1 -> Less Than4/2
  Add1/1 -> Abs1/1
  [VTQD_RollRegenDisableReq_flg] -> NOT/1
  [VTQD_RrTqErr_Nm] -> Less Than3/1
  Add/1 -> Abs/1
  [VTQD_BrkSwSta_flg] -> NOT3/1
  [VTQD_FrTqErr_Nm] -> Less Than4/1
  Abs1/1 -> [VTQD_FrTqErr_Nm]  "VTQD_FrTqErr_Nm"
  [VTQD_GearActualPosn_enum] -> Equal1/1
  [VINP_VehSpeed_kph] -> Less Than1/1
  [VINP_RegenMode_enum] -> Equal2/1
  [VTQD_AfterAvailableTqDemFr_Nm] -> Delay4/1
  Constant1/1 -> Less Than2/2
  [VTQD_AfterAvailableTqDemRr_Nm] -> Delay2/1
  Less Than4/1 -> AND1/8  "VTQD_VehWeightEstEnCon7_flg"
  [VINP_RrRBCActive_flg] -> NOT4/1
  [VTQR_NoABSREDUWhlTqReq_Nm] -> Delay3/1
  NOT/1 -> AND1/4  "VTQD_VehWeightEstEnCon4_flg"
  [VINP_FrRBCActive_flg] -> NOT5/1
  Constant5/1 -> Less Than5/2
  Equal2/1 -> AND1/5  "VTQD_VehWeightEstEnCon5_flg"
  [VTQD_LowIdleAccPedal_flg] -> AND1/6
  Constant2/1 -> Equal2/2
  Less Than3/1 -> AND1/7  "VTQD_VehWeightEstEnCon6_flg"
  Less Than2/1 -> AND1/3  "VTQD_VehWeightEstEnCon3_flg"
  [VINP_VehSpeed_kph] -> Less Than2/1
  Less Than5/1 -> AND1/12  "VTQD_VehWeightEstEnCon11_flg"
  [VINP_GRADE_Deg] -> Abs2/1
  Abs2/1 -> Less Than5/1
  Constant3/1 -> Less Than3/2
  VTQD_AfterAvailableTqDemRr_Nm/1 -> [VTQD_AfterAvailableTqDemRr_Nm]
  VTQR_NoABSREDUWhlTqReq_Nm/1 -> [VTQR_NoABSREDUWhlTqReq_Nm]
  VTQD_AfterAvailableTqDemFr_Nm/1 -> [VTQD_AfterAvailableTqDemFr_Nm]
  VTQR_NoABSFEDUWhlTqReq_Nm/1 -> [VTQR_NoABSFEDUWhlTqReq_Nm]
  VTQD_GearActualPosn_enum/1 -> [VTQD_GearActualPosn_enum]
  VINP_VehSpeed_kph/1 -> [VINP_VehSpeed_kph]
  VTQD_RollRegenDisableReq_flg/1 -> [VTQD_RollRegenDisableReq_flg]
  VINP_RegenMode_enum/1 -> [VINP_RegenMode_enum]
  VTQD_LowIdleAccPedal_flg/1 -> [VTQD_LowIdleAccPedal_flg]
  VTQD_BrkSwSta_flg/1 -> [VTQD_BrkSwSta_flg]
  VINP_RrRBCActive_flg/1 -> [VINP_RrRBCActive_flg]
  VINP_FrRBCActive_flg/1 -> [VINP_FrRBCActive_flg]
  VINP_GRADE_Deg/1 -> [VINP_GRADE_Deg]
  [VTQD_VehWeightEstEn_flg] -> VTQD_VehWeightEstEn_flg/1
  Relational Operator/1 -> [VTQD_VehWeightEstDis_flg]  "VTQD_VehWeightEstDis_flg"
  Timer/1 -> Relational Operator/1
  NOT1/1 -> Timer/2
  [VTQD_VehWeightEstEn_flg] -> NOT1/1, Timer/1
  Constant6/1 -> Relational Operator/2, Timer/4
  [VTQD_VehWeightEstDis_flg] -> VTQD_VehWeightEstDis_flg/1
  task_time_s/1 -> [task_time_s]
  AND1/1 -> DelayEnable/1
  DelayEnable/1 -> [VTQD_VehWeightEstEn_flg]  "VTQD_VehWeightEstEn_flg"
  [task_time_s] -> DelayEnable/3
  Constant7/1 -> DelayEnable/2
  [VTQD_VehWeightEstEnd_flg] -> Detect Increase/1
  Detect Increase/1 -> SR_Latch/1
  SR_Latch/1 -> NOT2/1, Timer1/1
  NOT2/1 -> Timer1/2
  Constant8/1 -> Relational Operator1/2, Timer1/4
  Timer1/1 -> [VTQD_EstVehWeightResetTime_s], Relational Operator1/1  "VTQD_EstVehWeightResetTime_s"
  Relational Operator1/1 -> [VTQD_EstVehWeitResetFinish_flg]  "VTQD_EstVehWeitResetFinish_flg"
  [VTQD_EstVehWeitResetFinish_flg] -> Delay/1
  Delay/1 -> SR_Latch/2
  [VTQD_EstVehWeightResetTime_s] -> Delay5/1
  Constant10/1 -> Equal/2
  Equal/1 -> AND1/13  "VTQD_VehWeightEstEnCon12_flg"
  VTQD_VehWeightEstEnd_flg/1 -> [VTQD_VehWeightEstEnd_flg]
  Delay1/1 -> Add1/1
  Delay2/1 -> Add/1
  Delay3/1 -> Add/2
  Delay4/1 -> Add1/2
  Delay5/1 -> Equal/1
  NOT3/1 -> AND1/9  "VTQD_VehWeightEstEnCon8_flg"
  NOT4/1 -> AND1/10  "VTQD_VehWeightEstEnCon9_flg"
  NOT5/1 -> AND1/11  "VTQD_VehWeightEstEnCon10_flg"
  [task_time_s] -> Timer/3
  [task_time_s] -> Timer1/3

== system tqdtqr_rebuild_V3/Input_Convert/Signal function/VehWeightEst/Desicion ==
  task_time_s : Inport
  VTQD_VehWeightEstDis_flg : Inport  Port=2
  VTQD_EstVehWeight_kg : Inport  Port=3
  VINP_DriverSeatBeltCmd_flg : Inport  Port=4
  VINP_PsngrSeatBeltCmd_flg : Inport  Port=5
  VINP_RDriverSeatBeltCmd_flg : Inport  Port=6
  VINP_RCenterSeatBeltCmd_flg : Inport  Port=7
  VINP_RPsngrSeatBeltCmd_flg : Inport  Port=8
  VTQD_EstLongAccCheckPass_flg : Inport  Port=9
  VTQD_EstFrRealTqCheckPass_flg : Inport  Port=10
  VTQD_EstRrRealTqCheckPass_flg : Inport  Port=11
  AND : Logic  Inputs=5  AllPortsSameDT=off  OutDataTypeStr=boolean
  Add : Sum  Inputs=+++++
  Constant1 : Constant  Value=eps
  Constant{2,4,6,8,10} (5 alike) : Constant  Value=ZERO_INT
  Constant{3,5,7,9,11} (5 alike) : Constant  Value=ONE_INT
  Constant12 : Constant  Value=KTQD_EstEndDelayTime_s
  Data Type Conversion : DataTypeConversion  OutDataTypeStr=single
  Delay : Delay  DelayLength=1  InitialCondition=boolean(0)
      settings: AttributesFormatString=%<InitialCondition>
  Delay1 : Delay  DelayLength=1  InitialCondition=single(0.0)
      settings: AttributesFormatString=%<InitialCondition>
  DelayEnable : hcu_lib/Basic_Blocks/DelayEnable
  Equal : RelationalOperator  OutDataTypeStr=boolean  RndMeth=Simplest
  MTQD_EstInitVehWeight_Y_kg : Lookup_n-D  NumberOfTableDimensions=1  BreakpointsForDimension1=ATQD_EstInitVehWeight_X_c  Table=MTQD_EstInitVehWeight_Y_kg  ExtrapMethod=Clip  InternalRulePriority=Speed  RndMeth=Simplest  InputSameDT=on
  NOT : Logic  Operator=NOT  AllPortsSameDT=off  OutDataTypeStr=boolean
  Switch{,1..6} (7 alike) : Switch  Criteria=u2 ~= 0
      settings: AttributesFormatString=%<Criteria>
  VTQD_VehWeightEstEnd_flg : Outport
  VTQD_EstVehWeightResult_kg : Outport  Port=2
  wires:
  Constant7/1 -> Switch4/1
  Constant1/1 -> Equal/2
  Switch2/1 -> Add/1
  [VINP_DriverSeatBeltCmd_flg] -> Switch2/2
  [VINP_RCenterSeatBeltCmd_flg] -> Switch4/2
  Switch5/1 -> Add/4
  Equal/1 -> Switch1/2
  Constant10/1 -> Switch6/3
  [VTQD_VehWeightEstDis_flg] -> AND/1
  Switch6/1 -> Add/5
  Delay/1 -> NOT/1
  Switch3/1 -> Add/2
  Constant6/1 -> Switch4/3
  Constant3/1 -> Switch2/1
  [VTQD_EstActVehWeight_kg] -> Switch1/1
  Constant2/1 -> Switch2/3
  [VTQD_VehWeightEstEnter_flg] -> Switch/2
  Constant11/1 -> Switch6/1
  Switch1/1 -> [VTQD_EstVehWeightResult_kg]  "VTQD_EstVehWeightResult_kg"
  Constant4/1 -> Switch3/3
  Constant5/1 -> Switch3/1
  [VINP_RDriverSeatBeltCmd_flg] -> Switch5/2
  Switch/1 -> Delay1/1, [VTQD_EstActVehWeight_kg]  "VTQD_EstActVehWeight_kg"
  AND/1 -> [VTQD_VehWeightEstEnter_flg]  "VTQD_VehWeightEstEnter_flg"
  [VINP_RPsngrSeatBeltCmd_flg] -> Switch6/2
  [VTQD_EstActVehWeight_kg] -> Equal/1
  [VINP_PsngrSeatBeltCmd_flg] -> Switch3/2
  Delay1/1 -> Switch/3
  [VTQD_EstInitVehWeight_kg] -> Switch1/3
  Constant9/1 -> Switch5/1
  Constant8/1 -> Switch5/3
  [VTQD_EstVehWeight_kg] -> Switch/1
  [VTQD_VehWeightEstEnd_flg] -> Delay/1
  NOT/1 -> AND/2
  Switch4/1 -> Add/3
  [VTQD_VehWeightEstDis_flg] -> DelayEnable/1
  Constant12/1 -> DelayEnable/2
  [task_time_s] -> DelayEnable/3
  DelayEnable/1 -> [VTQD_VehWeightEstEnd_flg]  "VTQD_VehWeightEstEnd_flg"
  task_time_s/1 -> [task_time_s]
  [VTQD_VehWeightEstEnd_flg] -> VTQD_VehWeightEstEnd_flg/1
  VTQD_VehWeightEstDis_flg/1 -> [VTQD_VehWeightEstDis_flg]
  VTQD_EstVehWeight_kg/1 -> [VTQD_EstVehWeight_kg]
  [VTQD_EstVehWeightResult_kg] -> VTQD_EstVehWeightResult_kg/1
  VINP_DriverSeatBeltCmd_flg/1 -> [VINP_DriverSeatBeltCmd_flg]
  VINP_PsngrSeatBeltCmd_flg/1 -> [VINP_PsngrSeatBeltCmd_flg]
  VINP_RDriverSeatBeltCmd_flg/1 -> [VINP_RDriverSeatBeltCmd_flg]
  VINP_RCenterSeatBeltCmd_flg/1 -> [VINP_RCenterSeatBeltCmd_flg]
  VINP_RPsngrSeatBeltCmd_flg/1 -> [VINP_RPsngrSeatBeltCmd_flg]
  VTQD_EstRrRealTqCheckPass_flg/1 -> [VTQD_EstRrRealTqCheckPass_flg]
  VTQD_EstFrRealTqCheckPass_flg/1 -> [VTQD_EstFrRealTqCheckPass_flg]
  VTQD_EstLongAccCheckPass_flg/1 -> [VTQD_EstLongAccCheckPass_flg]
  [VTQD_EstLongAccCheckPass_flg] -> AND/3
  [VTQD_EstFrRealTqCheckPass_flg] -> AND/4
  [VTQD_EstRrRealTqCheckPass_flg] -> AND/5
  MTQD_EstInitVehWeight_Y_kg/1 -> [VTQD_EstInitVehWeight_kg]  "VTQD_EstInitVehWeight_kg"
  Data Type Conversion/1 -> MTQD_EstInitVehWeight_Y_kg/1
  Add/1 -> Data Type Conversion/1  "VTQD_EstInitVehWightX_c"

== system tqdtqr_rebuild_V3/Input_Convert/Signal function/combo key/Combo Key Detection ==
  TASK_TIME_10_MS : Inport
  VSCP_ComboKeyEn_flg : Inport  Port=2
  VSCP_ComboKeyReset_flg : Inport  Port=3
  VSCP_ComboKey_enum : Inport  Port=4
  VSCP_ComboKeyEnter_flg : Inport  Port=5
  VSCP_StreetFightModeOff_flg : Inport  Port=6
  DiagnosisOff Mode : Subsystem
  Engineering Mode : Subsystem
  Exhibition Mode : Subsystem
  Manufacture Mode : Subsystem
  Street Fight Mode : Subsystem
  VSCP_StreetFightMode_flg : Outport
  VSCP_EngineeringMode_flg : Outport  Port=2
  VSCP_ManufactureMode_flg : Outport  Port=3
  VSCP_ExhibitionMode_flg : Outport  Port=4
  VSCP_DiagnosisOffMode_flg : Outport  Port=5
  wires:
  [VSCP_ComboKeyEn_flg] -> Street Fight Mode/2(VSCP_ComboKeyEn_flg)
  [VSCP_StreetFightModeOff_flg] -> Street Fight Mode/6(VSCP_StreetFightModeOff_flg)
  Street Fight Mode/1(VSCP_StreetFightMode_flg) -> [VSCP_StreetFightMode_flg]
  [VSCP_ComboKeyReset_flg] -> Street Fight Mode/3(VSCP_ComboKeyReset_flg)
  [TASK_TIME_10_MS] -> Street Fight Mode/1(TASK_TIME_10_MS)
  [VSCP_ComboKeyEnter_flg] -> Street Fight Mode/5(VSCP_ComboKeyEnter_flg)
  [VSCP_ComboKey_enum] -> Street Fight Mode/4(VSCP_ComboKey_enum)
  TASK_TIME_10_MS/1 -> [TASK_TIME_10_MS]
  VSCP_ComboKeyEn_flg/1 -> [VSCP_ComboKeyEn_flg]
  VSCP_ComboKeyReset_flg/1 -> [VSCP_ComboKeyReset_flg]
  VSCP_ComboKey_enum/1 -> [VSCP_ComboKey_enum]
  VSCP_ComboKeyEnter_flg/1 -> [VSCP_ComboKeyEnter_flg]
  VSCP_StreetFightModeOff_flg/1 -> [VSCP_StreetFightModeOff_flg]
  [VSCP_ComboKey_enum] -> Engineering Mode/4(VSCP_ComboKey_enum)
  [VSCP_ComboKeyEnter_flg] -> Engineering Mode/5(VSCP_ComboKeyEnter_flg)
  [TASK_TIME_10_MS] -> Engineering Mode/1(TASK_TIME_10_MS)
  [VSCP_ComboKeyReset_flg] -> Engineering Mode/3(VSCP_ComboKeyReset_flg)
  Engineering Mode/1(VSCP_EngineeringMode_flg) -> [VSCP_EngineeringMode_flg]
  [VSCP_StreetFightModeOff_flg] -> Engineering Mode/6(VSCP_StreetFightModeOff_flg)
  [VSCP_ComboKeyEn_flg] -> Engineering Mode/2(VSCP_ComboKeyEn_flg)
  [VSCP_StreetFightMode_flg] -> VSCP_StreetFightMode_flg/1
  [VSCP_EngineeringMode_flg] -> VSCP_EngineeringMode_flg/1
  [VSCP_ComboKeyEn_flg] -> Manufacture Mode/2(VSCP_ComboKeyEn_flg)
  [VSCP_StreetFightModeOff_flg] -> Manufacture Mode/6(VSCP_StreetFightModeOff_flg)
  [VSCP_ComboKeyReset_flg] -> Manufacture Mode/3(VSCP_ComboKeyReset_flg)
  [TASK_TIME_10_MS] -> Manufacture Mode/1(TASK_TIME_10_MS)
  [VSCP_ComboKeyEnter_flg] -> Manufacture Mode/5(VSCP_ComboKeyEnter_flg)
  [VSCP_ComboKey_enum] -> Manufacture Mode/4(VSCP_ComboKey_enum)
  Manufacture Mode/1(VSCP_ManufactureMode_flg) -> [VSCP_ManufactureMode_flg]
  [VSCP_ComboKey_enum] -> Exhibition Mode/4(VSCP_ComboKey_enum)
  [VSCP_ComboKeyEnter_flg] -> Exhibition Mode/5(VSCP_ComboKeyEnter_flg)
  [TASK_TIME_10_MS] -> Exhibition Mode/1(TASK_TIME_10_MS)
  [VSCP_ComboKeyReset_flg] -> Exhibition Mode/3(VSCP_ComboKeyReset_flg)
  [VSCP_StreetFightModeOff_flg] -> Exhibition Mode/6(VSCP_StreetFightModeOff_flg)
  [VSCP_ComboKeyEn_flg] -> Exhibition Mode/2(VSCP_ComboKeyEn_flg)
  Exhibition Mode/1(VSCP_ExhibitionMode_flg) -> [VSCP_ExhibitionMode_flg]
  [VSCP_ManufactureMode_flg] -> VSCP_ManufactureMode_flg/1
  [VSCP_ExhibitionMode_flg] -> VSCP_ExhibitionMode_flg/1
  [VSCP_ComboKeyEn_flg] -> DiagnosisOff Mode/2(VSCP_ComboKeyEn_flg)
  [VSCP_StreetFightModeOff_flg] -> DiagnosisOff Mode/6(VSCP_StreetFightModeOff_flg)
  [VSCP_ComboKeyReset_flg] -> DiagnosisOff Mode/3(VSCP_ComboKeyReset_flg)
  [TASK_TIME_10_MS] -> DiagnosisOff Mode/1(TASK_TIME_10_MS)
  [VSCP_ComboKeyEnter_flg] -> DiagnosisOff Mode/5(VSCP_ComboKeyEnter_flg)
  [VSCP_ComboKey_enum] -> DiagnosisOff Mode/4(VSCP_ComboKey_enum)
  DiagnosisOff Mode/1(VSCP_DiagnosisOffMode_flg) -> [VSCP_DiagnosisOffMode_flg]
  [VSCP_DiagnosisOffMode_flg] -> VSCP_DiagnosisOffMode_flg/1
